simulink model "EngineSpeed_harness"  (Simulink 7.7)
settings: Solver=FixedStepDiscrete  SolverMode=SingleTasking  StartTime=0.0  StopTime=100  FixedStep=.01  RelTol=1e-3
InitFcn:
  | if signalbuilder('EngineSpeed_harness/Signal_Builder','activegroup') == 1
  |   CD_ENGINE_SPEED_FUNCTION.DataType = 'uint8';
  |   CD_ENGINE_SPEED_FUNCTION.Value = 255;
  | else
  |   CD_ENGINE_SPEED_FUNCTION.DataType = 'uint8';
  |   CD_ENGINE_SPEED_FUNCTION.Value = 0;
  | end
  | 
  | if signalbuilder('EngineSpeed_harness/Signal_Builder','activegroup') == 4
  |   CD_SHUTDOWN_FUNCTION.DataType = 'uint8';
  |   CD_SHUTDOWN_FUNCTION.Value = 255;
  | else
  |   CD_SHUTDOWN_FUNCTION.DataType = 'uint8';
  |   CD_SHUTDOWN_FUNCTION.Value = 0;
  | end
  | 
  | if signalbuilder('EngineSpeed_harness/Signal_Builder','activegroup') == 6
  |   CD_EOP_FUNCTION.DataType = 'uint8';
  |   CD_EOP_FUNCTION.Value = 0;
  | else
  |   CD_EOP_FUNCTION.DataType = 'uint8';
  |   CD_EOP_FUNCTION.Value = 1;
  | end
  | 
  | if (signalbuilder('EngineSpeed_harness/Signal_Builder','activegroup') == 6 || signalbuilder('EngineSpeed_harness/Signal_Builder','activegroup') == 7)
  |   CD_ENGINE_SPEED_DEBOUNCE_NO_SIGNAL.DataType = 'uint16';
  |   CD_ENGINE_SPEED_DEBOUNCE_NO_SIGNAL.Value = 100;
  |   CD_ENGINE_SPEED_DEBOUNCE_NORMAL.DataType = 'uint16';
  |   CD_ENGINE_SPEED_DEBOUNCE_NORMAL.Value = 50;
  | else
  |   CD_ENGINE_SPEED_DEBOUNCE_NO_SIGNAL.DataType = 'uint16';
  |   CD_ENGINE_SPEED_DEBOUNCE_NO_SIGNAL.Value = 3000;
  |   CD_ENGINE_SPEED_DEBOUNCE_NORMAL.DataType = 'uint16';
  |   CD_ENGINE_SPEED_DEBOUNCE_NORMAL.Value = 500;
  | end
  | 
  | if signalbuilder('EngineSpeed_harness/Signal_Builder','activegroup') == 9
  |   CD_ECU_FUNCTION.DataType = 'uint8';
  |   CD_ECU_FUNCTION.Value = 0;
  | else
  |   CD_ECU_FUNCTION.DataType = 'uint8';
  |   CD_ECU_FUNCTION.Value = 255;
  | end
  | 
  | if signalbuilder('EngineSpeed_harness/Signal_Builder','activegroup') == 14
  |   CD_ECU_FUNCTION.DataType = 'uint8';
  |   CD_ECU_FUNCTION.Value = 1;
  | end
undefined symbols (not defined in the file): CD_ENGINE_RPM_FACTOR, CD_ENGINE_SPEED_FILTER_FAST_VALUE, CD_ENGINE_SPEED_FILTER_SLOW_VALUE, CD_ENGINE_SPEED_RUNNING, CD_FLYWHEEL_TEETH, NON_FUNCTIONAL, PERIOD_COUNTS_PER_SECOND, sigbuilder_block, srate
libraries: simulink x2
CloseFcn:
  | rtwprivate ssgencode ModelCloseRequest sle_main_controller
settings Model: Creator=spencermindeman  LastModifiedBy=aliebel  CovMetricSettings=dcmw  CovForceBlockReductionOff=off  CovModelRefEnable=off
settings MATStruct: SampleTime=0.01  Offset=0  Priority=[1.0]
settings DataIOCC: LimitDataPoints=off  SaveOutput=off  SaveTime=off
settings OptimizationCC: BlockReduction=off  InlineParams=on  ExpressionFolding=off  StateBitsets=on  DataBitsets=on  UseTempVars=on  InitFltsAndDblsToZero=on  NoFixptDivByZeroProtection=on  EfficientFloat2IntCast=on  OptimizeModelRefInitCode=on
settings DebuggingCC: SaveWithParameterizedLinksMsg=none  MultiTaskDSMMsg=warning  MultiTaskCondExecSysMsg=none  IntegerOverflowMsg=none  ModelReferenceCSMismatchMessage=warning
settings HardwareCC: ProdBitPerInt=16  ProdBitPerPointer=16  ProdIntDivRoundTo=Floor  ProdEndianess=BigEndian  ProdWordSize=16  ProdHWDeviceType=Motorola HC12
settings ModelReferenceCC: ModelReferenceNumInstancesAllowed=Single
settings RTWCC: SystemTargetFile=ert.tlc  GenCodeOnly=on  TemplateMakefile=ert_default_tmf  Description=Real-Time Workshop Embedded Coder (no auto configuration)  GenerateReport=on  RetainRTWFile=on  ProcessScript=ert_make_rtw_hook  IncludeHyperlinkInReport=on  LaunchReport=on  IncludeERTFirstTime=on
settings RTWCC: CustomHeaderCode=|
  | #include "cpp_req_defines.h"
  | #include "hw_fin.h"
  | #include "cdata.h"
settings CodeAppCC: IgnoreCustomStorageClasses=off  DefineNamingRule=UpperCase
settings ERTTargetCC: TargetFcnLib=ansi_tfl_tmw.mat  FunctionExecutionProfile=off  MultiwordLength=2048  GenerateSampleERTMain=on  IncludeMdlTerminateFcn=off  SupportAbsoluteTime=off  SupportNonFinite=off  SupportComplex=off  PurelyIntegerCode=on  ERTCustomFileTemplate=gen_rtw_req_defines_h.tlc  GlobalDataDefinition=InSeparateSourceFile  GlobalDataReference=InSeparateHeaderFile  ConvertIfToSwitch=off

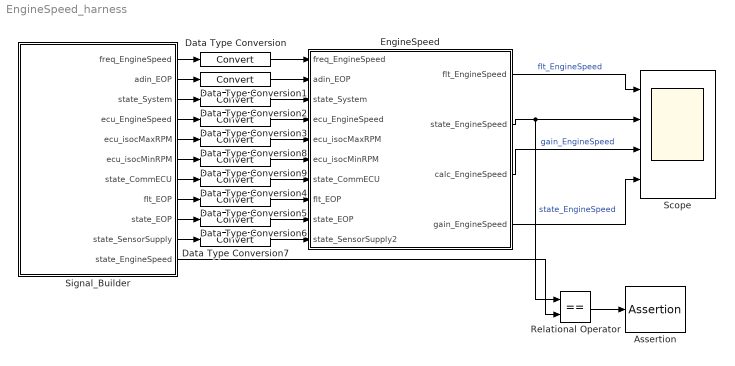
== system EngineSpeed_harness ==
  Assertion : Assertion  Enabled=off
  Data Type Conversion{,1..9} (10 alike) : DataTypeConversion
  EngineSpeed : Subsystem  TreatAsAtomicUnit=on  SystemSampleTime=srate  RTWFileName=mod_Inputs
      settings: RTWSystemCode=Function  RTWFcnNameOpts=Use subsystem name  RTWFileNameOpts=User specified
  Relational Operator : RelationalOperator  Operator===  OutDataTypeStr=boolean
  Scope : Scope  NumInputPorts=4
      settings: YMin=0~8~30~0  YMax=30~13~30~4  MaxDataPoints=50000
  Signal_Builder : Subsystem  Tag=STV Subsys  LoadFcn=sigbuilder_block('load');  StartFcn=sigbuilder_block('start');  StopFcn=sigbuilder_block('stop');  ClipboardFcn=sigbuilder_block('clipboard');  mask(Sigbuilder block){}
      mask help: Sigbuilder GUI
      mask init:
      | if ~strcmp(get_param(bdroot(gcbh),'SimulationStatus'),'stopped') tuvar = sigbuilder_block('maskInit'); end
      settings: CopyFcn=sigbuilder_block('copy');  DeleteFcn=sigbuilder_block('delete');  ModelCloseFcn=sigbuilder_block('modelClose');  PreSaveFcn=sigbuilder_block('preSave');  NameChangeFcn=sigbuilder_block('namechange');  OpenFcn=sigbuilder_block('open',[39.75 48.75 1278 690.75 ]);  CloseFcn=sigbuilder_block('close');
      mask Display: plot(0,0,100,100,[10,10,40,40,10],[80,20,20,80,80],[40,10],[50,50], [40,27,10],[65,72,56],[40,25,25,10],[28,28,43,43]);
  wires:
  Data Type Conversion/1 -> EngineSpeed/1(freq_EngineSpeed)
  Data Type Conversion1/1 -> EngineSpeed/2(adin_EOP)
  Data Type Conversion2/1 -> EngineSpeed/3(state_System)
  Signal_Builder/1(freq_EngineSpeed) -> Data Type Conversion/1
  Data Type Conversion3/1 -> EngineSpeed/4(ecu_EngineSpeed)
  Relational Operator/1 -> Assertion/1
  Signal_Builder/11(state_EngineSpeed) -> Relational Operator/2
  Data Type Conversion4/1 -> EngineSpeed/7(state_CommECU)
  Signal_Builder/2(adin_EOP) -> Data Type Conversion1/1
  Signal_Builder/3(state_System) -> Data Type Conversion2/1
  Signal_Builder/4(ecu_EngineSpeed) -> Data Type Conversion3/1
  Signal_Builder/7(state_CommECU) -> Data Type Conversion4/1
  Signal_Builder/8(flt_EOP) -> Data Type Conversion5/1
  Signal_Builder/9(state_EOP) -> Data Type Conversion6/1
  Data Type Conversion5/1 -> EngineSpeed/8(flt_EOP)
  Data Type Conversion6/1 -> EngineSpeed/9(state_EOP)
  EngineSpeed/1(flt_EngineSpeed) -> Scope/1  "flt_EngineSpeed"
  EngineSpeed/2(state_EngineSpeed) -> Scope/2, Relational Operator/1  "state_EngineSpeed"
  EngineSpeed/3(calc_EngineSpeed) -> Scope/3  "gain_EngineSpeed"
  Signal_Builder/10(state_SensorSupply) -> Data Type Conversion7/1
  Data Type Conversion7/1 -> EngineSpeed/10(state_SensorSupply2)
  EngineSpeed/4(gain_EngineSpeed) -> Scope/4
  Signal_Builder/5(ecu_isocMaxRPM) -> Data Type Conversion8/1
  Signal_Builder/6(ecu_isocMinRPM) -> Data Type Conversion9/1
  Data Type Conversion8/1 -> EngineSpeed/5(ecu_isocMaxRPM)
  Data Type Conversion9/1 -> EngineSpeed/6(ecu_isocMinRPM)

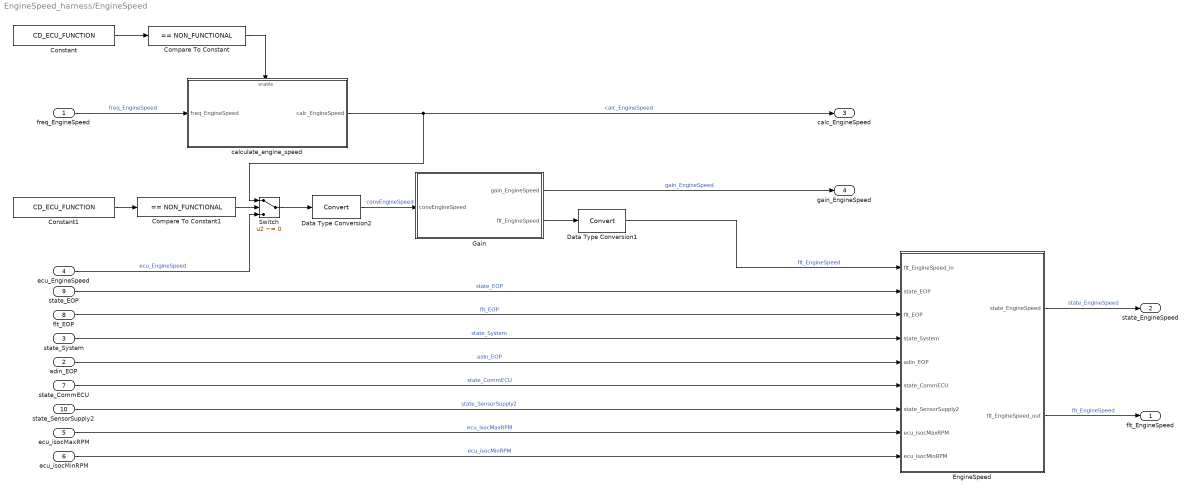
== system EngineSpeed_harness/EngineSpeed ==
  freq_EngineSpeed : Inport
  adin_EOP : Inport  Port=2
  state_System : Inport  Port=3
  ecu_EngineSpeed : Inport  Port=4
  ecu_isocMaxRPM : Inport  Port=5
  ecu_isocMinRPM : Inport  Port=6
  state_CommECU : Inport  Port=7
  flt_EOP : Inport  Port=8
  state_EOP : Inport  Port=9
  state_SensorSupply2 : Inport  Port=10
  Compare To Constant : simulink/Logic and Bit Operations/Compare To Constant  SystemSampleTime=-1  relop===  const=NON_FUNCTIONAL  LogicOutDataTypeMode=boolean  ZeroCross=off
  Compare To Constant1 : simulink/Logic and Bit Operations/Compare To Constant  SystemSampleTime=-1  relop===  const=NON_FUNCTIONAL  LogicOutDataTypeMode=boolean  ZeroCross=off
  Constant : Constant  Value=CD_ECU_FUNCTION  OutDataTypeStr=uint8
  Constant1 : Constant  Value=CD_ECU_FUNCTION  OutDataTypeStr=uint8
  Data Type Conversion1 : DataTypeConversion
  Data Type Conversion2 : DataTypeConversion
  EngineSpeed : Stateflow chart  TreatAsAtomicUnit=on
  Gain : Stateflow chart  TreatAsAtomicUnit=on
  Switch : Switch  Criteria=u2 ~= 0
  calculate_engine_speed : Subsystem
  flt_EngineSpeed : Outport  OutDataTypeStr=uint16
  state_EngineSpeed : Outport  Port=2  OutDataTypeStr=uint8
  calc_EngineSpeed : Outport  Port=3  OutDataTypeStr=uint16
  gain_EngineSpeed : Outport  Port=4
  wires:
  adin_EOP/1 -> EngineSpeed/5(adin_EOP)  "adin_EOP"
  state_System/1 -> EngineSpeed/4(state_System)  "state_System"
  state_EOP/1 -> EngineSpeed/2(state_EOP)  "state_EOP"
  EngineSpeed/1(state_EngineSpeed) -> state_EngineSpeed/1  "state_EngineSpeed"
  flt_EOP/1 -> EngineSpeed/3(flt_EOP)  "flt_EOP"
  state_CommECU/1 -> EngineSpeed/6(state_CommECU)  "state_CommECU"
  freq_EngineSpeed/1 -> calculate_engine_speed/1(freq_EngineSpeed)  "freq_EngineSpeed"
  Data Type Conversion1/1 -> EngineSpeed/1(flt_EngineSpeed_in)  "flt_EngineSpeed"
  state_SensorSupply2/1 -> EngineSpeed/7(state_SensorSupply2)  "state_SensorSupply2"
  Gain/2(flt_EngineSpeed) -> Data Type Conversion1/1
  Data Type Conversion2/1 -> Gain/1(convEngineSpeed)  "convEngineSpeed"
  Gain/1(gain_EngineSpeed) -> gain_EngineSpeed/1  "gain_EngineSpeed"
  calculate_engine_speed/1(calc_EngineSpeed) -> Switch/1, calc_EngineSpeed/1  "calc_EngineSpeed"
  Switch/1 -> Data Type Conversion2/1
  Constant/1 -> Compare To Constant/1
  Compare To Constant/1 -> calculate_engine_speed/Enable
  Constant1/1 -> Compare To Constant1/1
  Compare To Constant1/1 -> Switch/2
  ecu_EngineSpeed/1 -> Switch/3  "ecu_EngineSpeed"
  EngineSpeed/2(flt_EngineSpeed_out) -> flt_EngineSpeed/1  "flt_EngineSpeed"
  ecu_isocMaxRPM/1 -> EngineSpeed/8(ecu_isocMaxRPM)  "ecu_isocMaxRPM"
  ecu_isocMinRPM/1 -> EngineSpeed/9(ecu_isocMinRPM)  "ecu_isocMinRPM"

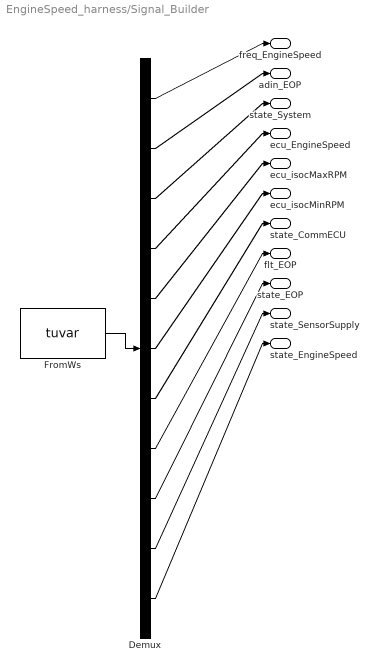
== system EngineSpeed_harness/Signal_Builder ==
  Demux : Demux  Tag=STV Demux  Outputs=11
  FromWs : FromWorkspace  Tag=STV FromWs  VariableName=tuvar  SampleTime=0  SigBuilderData=DataTag0  VnvData=DataTag1
      SigBuilderData=|
      | common.afterFinalStr = 'Extrapolate'
      | common.sampleTime = 0
      | dataSet(1).timeRange = [0 100]
      | dataSet(1).name = 'T1-NONFUNC'
      | dataSet(2).timeRange = [0 100]
      | dataSet(2).name = 'T2-NORMAL'
      | dataSet(3).timeRange = [0 100]
      | dataSet(3).name = 'T3-OOR'
      | dataSet(4).timeRange = [0 100]
      | dataSet(4).name = 'T4-EX HIGH'
      | dataSet(5).timeRange = [0 100]
      | dataSet(5).name = 'T5-Shutdown'
      | dataSet(6).timeRange = [0 100]
      | dataSet(6).name = 'T6-No Sig Sender'
      | dataSet(7).timeRange = [0 100]
      | dataSet(7).name = 'T7-No Sig Switch'
      | dataSet(8).timeRange = [0 100]
      | dataSet(8).name = 'T8-SystemState'
      | dataSet(9).timeRange = [0 100]
      | dataSet(9).name = 'T9-ECU'
      | dataSet(10).timeRange = [0 100]
      | dataSet(10).name = 'NORMAL1'
      | dataSet(11).timeRange = [0 100]
      | dataSet(11).name = 'NORMAL2'
      | dataSet(12).timeRange = [0 100]
      | dataSet(12).name = 'SystemState1'
      | dataSet(13).timeRange = [0 100]
      | dataSet(13).name = 'SystemState2'
      | dataSet(14).timeRange = [0 100]
      | dataSet(14).name = 'T14-ECU Invalid'
      | sbobj.Groups(1).Name = 'T1-NONFUNC'
      | sbobj.Groups(1).Signals(1).Name = 'freq_EngineSpeed'
      | sbobj.Groups(1).Signals(1).XData = [0 27.8 28.2 62.2 62.2 100]
      | sbobj.Groups(1).Signals(1).YData = [60000 60000 591 591 60500 60000]
      | sbobj.Groups(1).Signals(2).Name = 'adin_EOP'
      | sbobj.Groups(1).Signals(2).XData = [0 40 40 70 70 100]
      | sbobj.Groups(1).Signals(2).YData = [0 0 1000 1000 0 0]
      | sbobj.Groups(1).Signals(3).Name = 'state_System'
      | sbobj.Groups(1).Signals(3).XData = [0 100]
      | sbobj.Groups(1).Signals(3).YData = [1 1]
      | sbobj.Groups(1).Signals(4).Name = 'ecu_EngineSpeed'
      | sbobj.Groups(1).Signals(4).XData = [0 100]
      | sbobj.Groups(1).Signals(4).YData = [0 0]
      | sbobj.Groups(1).Signals(5).Name = 'ecu_isocMaxRPM'
      | sbobj.Groups(1).Signals(5).XData = [0 100]
      | sbobj.Groups(1).Signals(5).YData = [0 0]
      | sbobj.Groups(1).Signals(6).Name = 'ecu_isocMinRPM'
      | sbobj.Groups(1).Signals(6).XData = [0 100]
      | sbobj.Groups(1).Signals(6).YData = [0 0]
      | sbobj.Groups(1).Signals(7).Name = 'state_CommECU'
      | sbobj.Groups(1).Signals(7).XData = [0 100]
      | sbobj.Groups(1).Signals(7).YData = [0 0]
      | sbobj.Groups(1).Signals(8).Name = 'flt_EOP'
      | sbobj.Groups(1).Signals(8).XData = [0 18.2 18.2 19.4 19.4 21 21 32.6 32.6 33 33 36.6 36.6 48.4 48.4 100]
      | sbobj.Groups(1).Signals(8).YData = [0 0 25 25 0.5 0.5 25 25 0.5 0.5 25 25 0 0 25 25]
      | sbobj.Groups(1).Signals(9).Name = 'state_EOP'
      | sbobj.Groups(1).Signals(9).XData = [0 59.8 59.8 70.8 70.8 100]
      | sbobj.Groups(1).Signals(9).YData = [8 8 10 10 8 8]
      | sbobj.Groups(1).Signals(10).Name = 'state_SensorSupply'
      | sbobj.Groups(1).Signals(10).XData = [0 100]
      | sbobj.Groups(1).Signals(10).YData = [0 0]
      | sbobj.Groups(1).Signals(11).Name = 'state_EngineSpeed'
      | sbobj.Groups(1).Signals(11).XData = [0 100]
      | sbobj.Groups(1).Signals(11).YData = [8 8]
      | sbobj.Groups(2).Name = 'T2-NORMAL'
      | sbobj.Groups(2).Signals(1).Name = 'freq_EngineSpeed'
      | sbobj.Groups(2).Signals(1).XData = [0 39.7 100]
      | sbobj.Groups(2).Signals(1).YData = [1000 692 1000]
      | sbobj.Groups(2).Signals(2).Name = 'adin_EOP'
      | sbobj.Groups(2).Signals(2).XData = [0 100]
      | sbobj.Groups(2).Signals(2).YData = [0 0]
      | sbobj.Groups(2).Signals(3).Name = 'state_System'
      | sbobj.Groups(2).Signals(3).XData = [0 100]
      | sbobj.Groups(2).Signals(3).YData = [1 1]
      | sbobj.Groups(2).Signals(4).Name = 'ecu_EngineSpeed'
      | sbobj.Groups(2).Signals(4).XData = [0 100]
      | sbobj.Groups(2).Signals(4).YData = [0 0]
      | sbobj.Groups(2).Signals(5).Name = 'ecu_isocMaxRPM'
      | sbobj.Groups(2).Signals(5).XData = [0 100]
      | sbobj.Groups(2).Signals(5).YData = [0 0]
      | sbobj.Groups(2).Signals(6).Name = 'ecu_isocMinRPM'
      | sbobj.Groups(2).Signals(6).XData = [0 100]
      | sbobj.Groups(2).Signals(6).YData = [0 0]
      | sbobj.Groups(2).Signals(7).Name = 'state_CommECU'
      | sbobj.Groups(2).Signals(7).XData = [0 100]
      | sbobj.Groups(2).Signals(7).YData = [0 0]
      | sbobj.Groups(2).Signals(8).Name = 'flt_EOP'
      | sbobj.Groups(2).Signals(8).XData = [0 100]
      | sbobj.Groups(2).Signals(8).YData = [20 20]
      | sbobj.Groups(2).Signals(9).Name = 'state_EOP'
      | sbobj.Groups(2).Signals(9).XData = [0 100]
      | sbobj.Groups(2).Signals(9).YData = [8 8]
      | sbobj.Groups(2).Signals(10).Name = 'state_SensorSupply'
      | sbobj.Groups(2).Signals(10).XData = [0 100]
      | sbobj.Groups(2).Signals(10).YData = [8 8]
      | sbobj.Groups(2).Signals(11).Name = 'state_EngineSpeed'
      | sbobj.Groups(2).Signals(11).XData = [0 100]
      | sbobj.Groups(2).Signals(11).YData = [8 8]
      | sbobj.Groups(3).Name = 'T3-OOR'
      | sbobj.Groups(3).Signals(1).Name = 'freq_EngineSpeed'
      | sbobj.Groups(3).Signals(1).XData = [0 19.8 46.8 46.8 47.4 47.4 50.2 54.8 54.8 55 55 100]
      | sbobj.Groups(3).Signals(1).YData = [1000 1000 289.473684211 1020 980 247.368421053 200 198.152610442 1020 1020 196.546184739 180]
      | sbobj.Groups(3).Signals(2).Name = 'adin_EOP'
      | sbobj.Groups(3).Signals(2).XData = [0 100]
      | sbobj.Groups(3).Signals(2).YData = [0 0]
      | sbobj.Groups(3).Signals(3).Name = 'state_System'
      | sbobj.Groups(3).Signals(3).XData = [0 100]
      | sbobj.Groups(3).Signals(3).YData = [1 1]
      | sbobj.Groups(3).Signals(4).Name = 'ecu_EngineSpeed'
      | sbobj.Groups(3).Signals(4).XData = [0 100]
      | sbobj.Groups(3).Signals(4).YData = [0 0]
      | sbobj.Groups(3).Signals(5).Name = 'ecu_isocMaxRPM'
      | sbobj.Groups(3).Signals(5).XData = [0 100]
      | sbobj.Groups(3).Signals(5).YData = [0 0]
      | sbobj.Groups(3).Signals(6).Name = 'ecu_isocMinRPM'
      | sbobj.Groups(3).Signals(6).XData = [0 100]
      | sbobj.Groups(3).Signals(6).YData = [0 0]
      | sbobj.Groups(3).Signals(7).Name = 'state_CommECU'
      | sbobj.Groups(3).Signals(7).XData = [0 100]
      | sbobj.Groups(3).Signals(7).YData = [0 0]
      | sbobj.Groups(3).Signals(8).Name = 'flt_EOP'
      | sbobj.Groups(3).Signals(8).XData = [0 100]
      | sbobj.Groups(3).Signals(8).YData = [20 20]
      | sbobj.Groups(3).Signals(9).Name = 'state_EOP'
      | sbobj.Groups(3).Signals(9).XData = [0 100]
      | sbobj.Groups(3).Signals(9).YData = [8 8]
      | sbobj.Groups(3).Signals(10).Name = 'state_SensorSupply'
      | sbobj.Groups(3).Signals(10).XData = [0 100]
      | sbobj.Groups(3).Signals(10).YData = [8 8]
      | sbobj.Groups(3).Signals(11).Name = 'state_EngineSpeed'
      | sbobj.Groups(3).Signals(11).XData = [0 37.26 37.26 37.97 37.97 38.99 38.99 47.32 47.32 50.49 50.49 100]
      | sbobj.Groups(3).Signals(11).YData = [8 8 10 10 11 11 15 15 8 8 18 18]
      | sbobj.Groups(4).Name = 'T4-EX HIGH'
      | sbobj.Groups(4).Signals(1).Name = 'freq_EngineSpeed'
      | sbobj.Groups(4).Signals(1).XData = [0 29.6 40 40.2 40.2 40.3 40.3 45.9 45.9 46 46 49.6 49.6 49.7 49.7 51.9 51.9 52 52 53.8 53.8 54.6 55.6 55.6 64.7 64.7 64.8 64.8 79.8 100]
      | sbobj.Groups(4).Signals(1).YData = [1000 1000 550 550 800 800 500 500 800 800 500 500 420 420 500 500 400 400 500 500 490 490 490 420 420 740 680 420 420 420]
      | sbobj.Groups(4).Signals(2).Name = 'adin_EOP'
      | sbobj.Groups(4).Signals(2).XData = [0 100]
      | sbobj.Groups(4).Signals(2).YData = [0 0]
      | sbobj.Groups(4).Signals(3).Name = 'state_System'
      | sbobj.Groups(4).Signals(3).XData = [0 100]
      | sbobj.Groups(4).Signals(3).YData = [1 1]
      | sbobj.Groups(4).Signals(4).Name = 'ecu_EngineSpeed'
      | sbobj.Groups(4).Signals(4).XData = [0 100]
      | sbobj.Groups(4).Signals(4).YData = [0 0]
      | sbobj.Groups(4).Signals(5).Name = 'ecu_isocMaxRPM'
      | sbobj.Groups(4).Signals(5).XData = [0 100]
      | sbobj.Groups(4).Signals(5).YData = [0 0]
      | sbobj.Groups(4).Signals(6).Name = 'ecu_isocMinRPM'
      | sbobj.Groups(4).Signals(6).XData = [0 100]
      | sbobj.Groups(4).Signals(6).YData = [0 0]
      | sbobj.Groups(4).Signals(7).Name = 'state_CommECU'
      | sbobj.Groups(4).Signals(7).XData = [0 100]
      | sbobj.Groups(4).Signals(7).YData = [0 0]
      | sbobj.Groups(4).Signals(8).Name = 'flt_EOP'
      | sbobj.Groups(4).Signals(8).XData = [0 100]
      | sbobj.Groups(4).Signals(8).YData = [20 20]
      | sbobj.Groups(4).Signals(9).Name = 'state_EOP'
      | sbobj.Groups(4).Signals(9).XData = [0 100]
      | sbobj.Groups(4).Signals(9).YData = [8 8]
      | sbobj.Groups(4).Signals(10).Name = 'state_SensorSupply'
      | sbobj.Groups(4).Signals(10).XData = [0 100]
      | sbobj.Groups(4).Signals(10).YData = [8 8]
      | sbobj.Groups(4).Signals(11).Name = 'state_EngineSpeed'
      | sbobj.Groups(4).Signals(11).XData = [0 45.35 45.35 60.67 60.67 100]
      | sbobj.Groups(4).Signals(11).YData = [8 8 10 10 11 11]
      | sbobj.Groups(5).Name = 'T5-Shutdown'
      | sbobj.Groups(5).Signals(1).Name = 'freq_EngineSpeed'
      | sbobj.Groups(5).Signals(1).XData = [0 29.6 40 40.2 40.2 40.3 40.3 45.9 45.9 46 46 49.6 49.6 49.7 49.7 51.9 51.9 52 52 57.8 57.8 58.3 58.3 58.7 58.7 64.7 64.7 64.8 64.8 79.8 79.8 100]
      | sbobj.Groups(5).Signals(1).YData = [1000 1000 550 550 800 800 500 500 800 800 410 410 420 420 440 440 400 400 770 770 490 490 750 750 400 400 740 680 400 400 420 420]
      | sbobj.Groups(5).Signals(2).Name = 'adin_EOP'
      | sbobj.Groups(5).Signals(2).XData = [0 100]
      | sbobj.Groups(5).Signals(2).YData = [0 0]
      | sbobj.Groups(5).Signals(3).Name = 'state_System'
      | sbobj.Groups(5).Signals(3).XData = [0 100]
      | sbobj.Groups(5).Signals(3).YData = [1 1]
      | sbobj.Groups(5).Signals(4).Name = 'ecu_EngineSpeed'
      | sbobj.Groups(5).Signals(4).XData = [0 100]
      | sbobj.Groups(5).Signals(4).YData = [0 0]
      | sbobj.Groups(5).Signals(5).Name = 'ecu_isocMaxRPM'
      | sbobj.Groups(5).Signals(5).XData = [0 100]
      | sbobj.Groups(5).Signals(5).YData = [0 0]
      | sbobj.Groups(5).Signals(6).Name = 'ecu_isocMinRPM'
      | sbobj.Groups(5).Signals(6).XData = [0 100]
      | sbobj.Groups(5).Signals(6).YData = [0 0]
      | sbobj.Groups(5).Signals(7).Name = 'state_CommECU'
      | sbobj.Groups(5).Signals(7).XData = [0 100]
      | sbobj.Groups(5).Signals(7).YData = [0 0]
      | sbobj.Groups(5).Signals(8).Name = 'flt_EOP'
      | sbobj.Groups(5).Signals(8).XData = [0 100]
      | sbobj.Groups(5).Signals(8).YData = [20 20]
      | sbobj.Groups(5).Signals(9).Name = 'state_EOP'
      | sbobj.Groups(5).Signals(9).XData = [0 100]
      | sbobj.Groups(5).Signals(9).YData = [8 8]
      | sbobj.Groups(5).Signals(10).Name = 'state_SensorSupply'
      | sbobj.Groups(5).Signals(10).XData = [0 100]
      | sbobj.Groups(5).Signals(10).YData = [8 8]
      | sbobj.Groups(5).Signals(11).Name = 'state_EngineSpeed'
      | sbobj.Groups(5).Signals(11).XData = [0 45.35 45.35 51.04 51.04 57.04 57.04 63.78 63.78 74.84 74.84 100]
      | sbobj.Groups(5).Signals(11).YData = [8 8 10 10 11 11 8 8 11 11 15 15]
      | sbobj.Groups(6).Name = 'T6-No Sig Sender'
      | sbobj.Groups(6).Signals(1).Name = 'freq_EngineSpeed'
      | sbobj.Groups(6).Signals(1).XData = [0 82.4 82.4 100]
      | sbobj.Groups(6).Signals(1).YData = [60000 60000 3000 3000]
      | sbobj.Groups(6).Signals(2).Name = 'adin_EOP'
      | sbobj.Groups(6).Signals(2).XData = [0 100]
      | sbobj.Groups(6).Signals(2).YData = [0 0]
      | sbobj.Groups(6).Signals(3).Name = 'state_System'
      | sbobj.Groups(6).Signals(3).XData = [0 100]
      | sbobj.Groups(6).Signals(3).YData = [1 1]
      | sbobj.Groups(6).Signals(4).Name = 'ecu_EngineSpeed'
      | sbobj.Groups(6).Signals(4).XData = [0 100]
      | sbobj.Groups(6).Signals(4).YData = [0 0]
      | sbobj.Groups(6).Signals(5).Name = 'ecu_isocMaxRPM'
      | sbobj.Groups(6).Signals(5).XData = [0 100]
      | sbobj.Groups(6).Signals(5).YData = [0 0]
      | sbobj.Groups(6).Signals(6).Name = 'ecu_isocMinRPM'
      | sbobj.Groups(6).Signals(6).XData = [0 100]
      | sbobj.Groups(6).Signals(6).YData = [0 0]
      | sbobj.Groups(6).Signals(7).Name = 'state_CommECU'
      | sbobj.Groups(6).Signals(7).XData = [0 100]
      | sbobj.Groups(6).Signals(7).YData = [0 0]
      | sbobj.Groups(6).Signals(8).Name = 'flt_EOP'
      | sbobj.Groups(6).Signals(8).XData = [0 18.2 18.2 19.4 19.4 21 21 32.6 32.6 33 33 36.6 36.6 48.4 48.4 100]
      | sbobj.Groups(6).Signals(8).YData = [0 0 25 25 0.5 0.5 25 25 0.5 0.5 25 25 0 0 25 25]
      | sbobj.Groups(6).Signals(9).Name = 'state_EOP'
      | sbobj.Groups(6).Signals(9).XData = [0 45.8 45.8 49.3 49.3 59.8 59.8 70.8 70.8 100]
      | sbobj.Groups(6).Signals(9).YData = [8 8 10 10 8 8 10 10 8 8]
      | sbobj.Groups(6).Signals(10).Name = 'state_SensorSupply'
      | sbobj.Groups(6).Signals(10).XData = [0 69.2 69.2 75.4 75.4 79.8 79.8 81.8 81.8 100]
      | sbobj.Groups(6).Signals(10).YData = [8 8 22 22 8 8 22 22 8 8]
      | sbobj.Groups(6).Signals(11).Name = 'state_EngineSpeed'
      | sbobj.Groups(6).Signals(11).XData = [0 19.21 19.21 19.91 19.91 22.01 22.01 37.11 37.11 50.31 50.31 60.31 60.31 76.41 76.41 80.32 80.32 100]
      | sbobj.Groups(6).Signals(11).YData = [8 8 13 13 8 8 13 13 8 8 13 13 8 8 13 13 8 8]
      | sbobj.Groups(7).Name = 'T7-No Sig Switch'
      | sbobj.Groups(7).Signals(1).Name = 'freq_EngineSpeed'
      | sbobj.Groups(7).Signals(1).XData = [0 82.4 82.4 100]
      | sbobj.Groups(7).Signals(1).YData = [60000 60000 3000 3000]
      | sbobj.Groups(7).Signals(2).Name = 'adin_EOP'
      | sbobj.Groups(7).Signals(2).XData = [0 40 40 70 70 75.1 75.1 78.6 78.6 100]
      | sbobj.Groups(7).Signals(2).YData = [0 0 1000 1000 0 0 990 990 0 0]
      | sbobj.Groups(7).Signals(3).Name = 'state_System'
      | sbobj.Groups(7).Signals(3).XData = [0 100]
      | sbobj.Groups(7).Signals(3).YData = [1 1]
      | sbobj.Groups(7).Signals(4).Name = 'ecu_EngineSpeed'
      | sbobj.Groups(7).Signals(4).XData = [0 100]
      | sbobj.Groups(7).Signals(4).YData = [0 0]
      | sbobj.Groups(7).Signals(5).Name = 'ecu_isocMaxRPM'
      | sbobj.Groups(7).Signals(5).XData = [0 100]
      | sbobj.Groups(7).Signals(5).YData = [0 0]
      | sbobj.Groups(7).Signals(6).Name = 'ecu_isocMinRPM'
      | sbobj.Groups(7).Signals(6).XData = [0 100]
      | sbobj.Groups(7).Signals(6).YData = [0 0]
      | sbobj.Groups(7).Signals(7).Name = 'state_CommECU'
      | sbobj.Groups(7).Signals(7).XData = [0 100]
      | sbobj.Groups(7).Signals(7).YData = [0 0]
      | sbobj.Groups(7).Signals(8).Name = 'flt_EOP'
      | sbobj.Groups(7).Signals(8).XData = [0 18.2 18.2 19.4 19.4 21 21 32.6 32.6 33 33 36.6 36.6 48.4 48.4 100]
      | sbobj.Groups(7).Signals(8).YData = [0 0 25 25 0.5 0.5 25 25 0.5 0.5 25 25 0 0 25 25]
      | sbobj.Groups(7).Signals(9).Name = 'state_EOP'
      | sbobj.Groups(7).Signals(9).XData = [0 9.8 9.8 35.4 35.4 42.3 42.3 59.8 59.8 70.8 70.8 100]
      | sbobj.Groups(7).Signals(9).YData = [9 9 8 8 9 9 8 8 10 10 8 8]
      | sbobj.Groups(7).Signals(10).Name = 'state_SensorSupply'
      | sbobj.Groups(7).Signals(10).XData = [0 100]
      | sbobj.Groups(7).Signals(10).YData = [8 8]
      | sbobj.Groups(7).Signals(11).Name = 'state_EngineSpeed'
      | sbobj.Groups(7).Signals(11).XData = [0 43.31 43.31 60.31 60.31 76.11 76.11 79.11 79.11 100]
      | sbobj.Groups(7).Signals(11).YData = [8 8 13 13 8 8 13 13 8 8]
      | sbobj.Groups(8).Name = 'T8-SystemState'
      | sbobj.Groups(8).Signals(1).Name = 'freq_EngineSpeed'
      | sbobj.Groups(8).Signals(1).XData = [0 39.7 100]
      | sbobj.Groups(8).Signals(1).YData = [1000 692 1000]
      | sbobj.Groups(8).Signals(2).Name = 'adin_EOP'
      | sbobj.Groups(8).Signals(2).XData = [0 100]
      | sbobj.Groups(8).Signals(2).YData = [0 0]
      | sbobj.Groups(8).Signals(3).Name = 'state_System'
      | sbobj.Groups(8).Signals(3).XData = [0 14.8 14.8 49.8 49.8 70 70 100]
      | sbobj.Groups(8).Signals(3).YData = [0 0 1 1 0 0 1 1]
      | sbobj.Groups(8).Signals(4).Name = 'ecu_EngineSpeed'
      | sbobj.Groups(8).Signals(4).XData = [0 100]
      | sbobj.Groups(8).Signals(4).YData = [0 0]
      | sbobj.Groups(8).Signals(5).Name = 'ecu_isocMaxRPM'
      | sbobj.Groups(8).Signals(5).XData = [0 100]
      | sbobj.Groups(8).Signals(5).YData = [0 0]
      | sbobj.Groups(8).Signals(6).Name = 'ecu_isocMinRPM'
      | sbobj.Groups(8).Signals(6).XData = [0 100]
      | sbobj.Groups(8).Signals(6).YData = [0 0]
      | sbobj.Groups(8).Signals(7).Name = 'state_CommECU'
      | sbobj.Groups(8).Signals(7).XData = [0 100]
      | sbobj.Groups(8).Signals(7).YData = [0 0]
      | sbobj.Groups(8).Signals(8).Name = 'flt_EOP'
      | sbobj.Groups(8).Signals(8).XData = [0 100]
      | sbobj.Groups(8).Signals(8).YData = [20 20]
      | sbobj.Groups(8).Signals(9).Name = 'state_EOP'
      | sbobj.Groups(8).Signals(9).XData = [0 100]
      | sbobj.Groups(8).Signals(9).YData = [8 8]
      | sbobj.Groups(8).Signals(10).Name = 'state_SensorSupply'
      | sbobj.Groups(8).Signals(10).XData = [0 100]
      | sbobj.Groups(8).Signals(10).YData = [8 8]
      | sbobj.Groups(8).Signals(11).Name = 'state_EngineSpeed'
      | sbobj.Groups(8).Signals(11).XData = [0 100]
      | sbobj.Groups(8).Signals(11).YData = [8 8]
      | sbobj.Groups(9).Name = 'T9-ECU'
      | sbobj.Groups(9).Signals(1).Name = 'freq_EngineSpeed'
      | sbobj.Groups(9).Signals(1).XData = [0 39.7 100]
      | sbobj.Groups(9).Signals(1).YData = [1000 692 1000]
      | sbobj.Groups(9).Signals(2).Name = 'adin_EOP'
      | sbobj.Groups(9).Signals(2).XData = [0 100]
      | sbobj.Groups(9).Signals(2).YData = [0 0]
      | sbobj.Groups(9).Signals(3).Name = 'state_System'
      | sbobj.Groups(9).Signals(3).XData = [0 100]
      | sbobj.Groups(9).Signals(3).YData = [1 1]
      | sbobj.Groups(9).Signals(4).Name = 'ecu_EngineSpeed'
      | sbobj.Groups(9).Signals(4).XData = [0 50.1 100]
      | sbobj.Groups(9).Signals(4).YData = [0 3000 0]
      | sbobj.Groups(9).Signals(5).Name = 'ecu_isocMaxRPM'
      | sbobj.Groups(9).Signals(5).XData = [0 100]
      | sbobj.Groups(9).Signals(5).YData = [0 0]
      | sbobj.Groups(9).Signals(6).Name = 'ecu_isocMinRPM'
      | sbobj.Groups(9).Signals(6).XData = [0 100]
      | sbobj.Groups(9).Signals(6).YData = [0 0]
      | sbobj.Groups(9).Signals(7).Name = 'state_CommECU'
      | sbobj.Groups(9).Signals(7).XData = [0 43.6 43.6 55.1 55.1 100]
      | sbobj.Groups(9).Signals(7).YData = [8 8 4 4 8 8]
      | sbobj.Groups(9).Signals(8).Name = 'flt_EOP'
      | sbobj.Groups(9).Signals(8).XData = [0 43.2 43.2 54.3 54.3 100]
      | sbobj.Groups(9).Signals(8).YData = [20 20 4 4 20 20]
      | sbobj.Groups(9).Signals(9).Name = 'state_EOP'
      | sbobj.Groups(9).Signals(9).XData = [0 100]
      | sbobj.Groups(9).Signals(9).YData = [8 8]
      | sbobj.Groups(9).Signals(10).Name = 'state_SensorSupply'
      | sbobj.Groups(9).Signals(10).XData = [0 100]
      | sbobj.Groups(9).Signals(10).YData = [8 8]
      | sbobj.Groups(9).Signals(11).Name = 'state_EngineSpeed'
      | sbobj.Groups(9).Signals(11).XData = [0 100]
      | sbobj.Groups(9).Signals(11).YData = [8 8]
      | sbobj.Groups(10).Name = 'NORMAL1'
      | sbobj.Groups(10).Signals(1).Name = 'freq_EngineSpeed'
      | sbobj.Groups(10).Signals(1).XData = [0 0.01 0.02 0.03 0.04 0.05 0.06 0.07 0.08 0.09 0.1 0.11 ... (1841 elements, 1x1841)]
      | sbobj.Groups(10).Signals(1).YData = [1028 1028 1021 1027 1020 1022 1028 1021 1021 1030 1024 1036 ... (1841 elements, 1x1841)]
      | sbobj.Groups(10).Signals(2).Name = 'adin_EOP'
      | sbobj.Groups(10).Signals(2).XData = [0 100]
      | sbobj.Groups(10).Signals(2).YData = [0 0]
      | sbobj.Groups(10).Signals(3).Name = 'state_System'
      | sbobj.Groups(10).Signals(3).XData = [0 100]
      | sbobj.Groups(10).Signals(3).YData = [1 1]
      | sbobj.Groups(10).Signals(4).Name = 'ecu_EngineSpeed'
      | sbobj.Groups(10).Signals(4).XData = [0 100]
      | sbobj.Groups(10).Signals(4).YData = [0 0]
      | sbobj.Groups(10).Signals(5).Name = 'ecu_isocMaxRPM'
      | sbobj.Groups(10).Signals(5).XData = [0 100]
      | sbobj.Groups(10).Signals(5).YData = [0 0]
      | sbobj.Groups(10).Signals(6).Name = 'ecu_isocMinRPM'
      | sbobj.Groups(10).Signals(6).XData = [0 100]
      | sbobj.Groups(10).Signals(6).YData = [0 0]
      | sbobj.Groups(10).Signals(7).Name = 'state_CommECU'
      | sbobj.Groups(10).Signals(7).XData = [0 100]
      | sbobj.Groups(10).Signals(7).YData = [0 0]
      | sbobj.Groups(10).Signals(8).Name = 'flt_EOP'
      | sbobj.Groups(10).Signals(8).XData = [0 100]
      | sbobj.Groups(10).Signals(8).YData = [20 20]
      | sbobj.Groups(10).Signals(9).Name = 'state_EOP'
      | sbobj.Groups(10).Signals(9).XData = [0 100]
      | sbobj.Groups(10).Signals(9).YData = [8 8]
      | sbobj.Groups(10).Signals(10).Name = 'state_SensorSupply'
      | sbobj.Groups(10).Signals(10).XData = [0 100]
      | sbobj.Groups(10).Signals(10).YData = [8 8]
      | sbobj.Groups(10).Signals(11).Name = 'state_EngineSpeed'
      | sbobj.Groups(10).Signals(11).XData = [0 100]
      | sbobj.Groups(10).Signals(11).YData = [8 8]
      | sbobj.Groups(11).Name = 'NORMAL2'
      | sbobj.Groups(11).Signals(1).Name = 'freq_EngineSpeed'
      | sbobj.Groups(11).Signals(1).XData = [0 0.01 0.02 0.03 0.04 0.05 0.06 0.07 0.08 0.09 0.1 0.11 ... (7018 elements, 1x7018)]
      | sbobj.Groups(11).Signals(1).YData = [1552 1552 1471 1355 1387 1292 1313 1313 1227 1188 1163 1178 ... (7018 elements, 1x7018)]
      | sbobj.Groups(11).Signals(2).Name = 'adin_EOP'
      | sbobj.Groups(11).Signals(2).XData = [0 100]
      | sbobj.Groups(11).Signals(2).YData = [0 0]
      | sbobj.Groups(11).Signals(3).Name = 'state_System'
      | sbobj.Groups(11).Signals(3).XData = [0 100]
      | sbobj.Groups(11).Signals(3).YData = [1 1]
      | sbobj.Groups(11).Signals(4).Name = 'ecu_EngineSpeed'
      | sbobj.Groups(11).Signals(4).XData = [0 100]
      | sbobj.Groups(11).Signals(4).YData = [0 0]
      | sbobj.Groups(11).Signals(5).Name = 'ecu_isocMaxRPM'
      | sbobj.Groups(11).Signals(5).XData = [0 100]
      | sbobj.Groups(11).Signals(5).YData = [0 0]
      | sbobj.Groups(11).Signals(6).Name = 'ecu_isocMinRPM'
      | sbobj.Groups(11).Signals(6).XData = [0 100]
      | sbobj.Groups(11).Signals(6).YData = [0 0]
      | sbobj.Groups(11).Signals(7).Name = 'state_CommECU'
      | sbobj.Groups(11).Signals(7).XData = [0 100]
      | sbobj.Groups(11).Signals(7).YData = [0 0]
      | sbobj.Groups(11).Signals(8).Name = 'flt_EOP'
      | sbobj.Groups(11).Signals(8).XData = [0 100]
      | sbobj.Groups(11).Signals(8).YData = [20 20]
      | sbobj.Groups(11).Signals(9).Name = 'state_EOP'
      | sbobj.Groups(11).Signals(9).XData = [0 100]
      | sbobj.Groups(11).Signals(9).YData = [8 8]
      | sbobj.Groups(11).Signals(10).Name = 'state_SensorSupply'
      | sbobj.Groups(11).Signals(10).XData = [0 100]
      | sbobj.Groups(11).Signals(10).YData = [8 8]
      | sbobj.Groups(11).Signals(11).Name = 'state_EngineSpeed'
      | sbobj.Groups(11).Signals(11).XData = [0 100]
      | sbobj.Groups(11).Signals(11).YData = [8 8]
      | sbobj.Groups(12).Name = 'SystemState1'
      | sbobj.Groups(12).Signals(1).Name = 'freq_EngineSpeed'
      | sbobj.Groups(12).Signals(1).XData = [0 0.02 0.04 0.06 0.08 0.1 0.12 0.14 0.16 0.18 0.2 0.22 ... (5001 elements, 1x5001)]
      | sbobj.Groups(12).Signals(1).YData = [1188 1163 1178 1131 1129 1111 1118 1123 1112 1130 1144 1155 ... (5001 elements, 1x5001)]
      | sbobj.Groups(12).Signals(2).Name = 'adin_EOP'
      | sbobj.Groups(12).Signals(2).XData = [0 100]
      | sbobj.Groups(12).Signals(2).YData = [0 0]
      | sbobj.Groups(12).Signals(3).Name = 'state_System'
      | sbobj.Groups(12).Signals(3).XData = [0 100]
      | sbobj.Groups(12).Signals(3).YData = [1 1]
      | sbobj.Groups(12).Signals(4).Name = 'ecu_EngineSpeed'
      | sbobj.Groups(12).Signals(4).XData = [0 100]
      | sbobj.Groups(12).Signals(4).YData = [0 0]
      | sbobj.Groups(12).Signals(5).Name = 'ecu_isocMaxRPM'
      | sbobj.Groups(12).Signals(5).XData = [0 100]
      | sbobj.Groups(12).Signals(5).YData = [0 0]
      | sbobj.Groups(12).Signals(6).Name = 'ecu_isocMinRPM'
      | sbobj.Groups(12).Signals(6).XData = [0 100]
      | sbobj.Groups(12).Signals(6).YData = [0 0]
      | sbobj.Groups(12).Signals(7).Name = 'state_CommECU'
      | sbobj.Groups(12).Signals(7).XData = [0 100]
      | sbobj.Groups(12).Signals(7).YData = [0 0]
      | sbobj.Groups(12).Signals(8).Name = 'flt_EOP'
      | sbobj.Groups(12).Signals(8).XData = [0 100]
      | sbobj.Groups(12).Signals(8).YData = [20 20]
      | sbobj.Groups(12).Signals(9).Name = 'state_EOP'
      | sbobj.Groups(12).Signals(9).XData = [0 100]
      | sbobj.Groups(12).Signals(9).YData = [8 8]
      | sbobj.Groups(12).Signals(10).Name = 'state_SensorSupply'
      | sbobj.Groups(12).Signals(10).XData = [0 100]
      | sbobj.Groups(12).Signals(10).YData = [8 8]
      | sbobj.Groups(12).Signals(11).Name = 'state_EngineSpeed'
      | sbobj.Groups(12).Signals(11).XData = [0 100]
      | sbobj.Groups(12).Signals(11).YData = [8 8]
      | sbobj.Groups(13).Name = 'SystemState2'
      | sbobj.Groups(13).Signals(1).Name = 'freq_EngineSpeed'
      | sbobj.Groups(13).Signals(1).XData = [0 0.01 0.02 0.03 0.04 0.05 0.06 0.07 0.08 0.09 0.1 0.11 ... (7012 elements, 1x7012)]
      | sbobj.Groups(13).Signals(1).YData = [1188 1163 1178 1131 1129 1111 1118 1123 1112 1130 1144 1155 ... (7012 elements, 1x7012)]
      | sbobj.Groups(13).Signals(2).Name = 'adin_EOP'
      | sbobj.Groups(13).Signals(2).XData = [0 100]
      | sbobj.Groups(13).Signals(2).YData = [0 0]
      | sbobj.Groups(13).Signals(3).Name = 'state_System'
      | sbobj.Groups(13).Signals(3).XData = [0 100]
      | sbobj.Groups(13).Signals(3).YData = [1 1]
      | sbobj.Groups(13).Signals(4).Name = 'ecu_EngineSpeed'
      | sbobj.Groups(13).Signals(4).XData = [0 100]
      | sbobj.Groups(13).Signals(4).YData = [0 0]
      | sbobj.Groups(13).Signals(5).Name = 'ecu_isocMaxRPM'
      | sbobj.Groups(13).Signals(5).XData = [0 100]
      | sbobj.Groups(13).Signals(5).YData = [0 0]
      | sbobj.Groups(13).Signals(6).Name = 'ecu_isocMinRPM'
      | sbobj.Groups(13).Signals(6).XData = [0 100]
      | sbobj.Groups(13).Signals(6).YData = [0 0]
      | sbobj.Groups(13).Signals(7).Name = 'state_CommECU'
      | sbobj.Groups(13).Signals(7).XData = [0 100]
      | sbobj.Groups(13).Signals(7).YData = [0 0]
      | sbobj.Groups(13).Signals(8).Name = 'flt_EOP'
      | sbobj.Groups(13).Signals(8).XData = [0 100]
      | sbobj.Groups(13).Signals(8).YData = [20 20]
      | sbobj.Groups(13).Signals(9).Name = 'state_EOP'
      | sbobj.Groups(13).Signals(9).XData = [0 100]
      | sbobj.Groups(13).Signals(9).YData = [8 8]
      | sbobj.Groups(13).Signals(10).Name = 'state_SensorSupply'
      | sbobj.Groups(13).Signals(10).XData = [0 100]
      | sbobj.Groups(13).Signals(10).YData = [8 8]
      | sbobj.Groups(13).Signals(11).Name = 'state_EngineSpeed'
      | sbobj.Groups(13).Signals(11).XData = [0 100]
      | sbobj.Groups(13).Signals(11).YData = [8 8]
      | sbobj.Groups(14).Name = 'T14-ECU Invalid'
      | sbobj.Groups(14).Signals(1).Name = 'freq_EngineSpeed'
      | sbobj.Groups(14).Signals(1).XData = [0 39.7 100]
      | sbobj.Groups(14).Signals(1).YData = [1000 692 1000]
      | sbobj.Groups(14).Signals(2).Name = 'adin_EOP'
      | sbobj.Groups(14).Signals(2).XData = [0 100]
      | sbobj.Groups(14).Signals(2).YData = [0 0]
      | sbobj.Groups(14).Signals(3).Name = 'state_System'
      | sbobj.Groups(14).Signals(3).XData = [0 100]
      | sbobj.Groups(14).Signals(3).YData = [1 1]
      | sbobj.Groups(14).Signals(4).Name = 'ecu_EngineSpeed'
      | sbobj.Groups(14).Signals(4).XData = [0 50.1 100]
      | sbobj.Groups(14).Signals(4).YData = [0 3000 0]
      | sbobj.Groups(14).Signals(5).Name = 'ecu_isocMaxRPM'
      | sbobj.Groups(14).Signals(5).XData = [0 1 1 5 5 6 6 11.1 11.1 14 14 17.7 17.7 21.9 21.9 23.8 23.8 100]
      | sbobj.Groups(14).Signals(5).YData = [2500 2500 1900 1900 2500 2500 1900 1900 2500 2500 3100 3100 2500 2500 3100 3100 2500 2500]
      | sbobj.Groups(14).Signals(6).Name = 'ecu_isocMinRPM'
      | sbobj.Groups(14).Signals(6).XData = [0 100]
      | sbobj.Groups(14).Signals(6).YData = [1000 1000]
      | sbobj.Groups(14).Signals(7).Name = 'state_CommECU'
      | sbobj.Groups(14).Signals(7).XData = [0 12 12 13 13 100]
      | sbobj.Groups(14).Signals(7).YData = [8 8 4 4 8 8]
      | sbobj.Groups(14).Signals(8).Name = 'flt_EOP'
      | sbobj.Groups(14).Signals(8).XData = [0 43.2 43.2 54.3 54.3 100]
      | sbobj.Groups(14).Signals(8).YData = [20 20 4 4 20 20]
      | sbobj.Groups(14).Signals(9).Name = 'state_EOP'
      | sbobj.Groups(14).Signals(9).XData = [0 100]
      | sbobj.Groups(14).Signals(9).YData = [8 8]
      | sbobj.Groups(14).Signals(10).Name = 'state_SensorSupply'
      | sbobj.Groups(14).Signals(10).XData = [0 100]
      | sbobj.Groups(14).Signals(10).YData = [8 8]
      | sbobj.Groups(14).Signals(11).Name = 'state_EngineSpeed'
      | sbobj.Groups(14).Signals(11).XData = [0 100]
      | sbobj.Groups(14).Signals(11).YData = [8 8]
  freq_EngineSpeed : Outport  Tag=STV Outport
  adin_EOP : Outport  Tag=STV Outport  Port=2
  state_System : Outport  Tag=STV Outport  Port=3
  ecu_EngineSpeed : Outport  Tag=STV Outport  Port=4
  ecu_isocMaxRPM : Outport  Tag=STV Outport  Port=5
  ecu_isocMinRPM : Outport  Tag=STV Outport  Port=6
  state_CommECU : Outport  Tag=STV Outport  Port=7
  flt_EOP : Outport  Tag=STV Outport  Port=8
  state_EOP : Outport  Tag=STV Outport  Port=9
  state_SensorSupply : Outport  Tag=STV Outport  Port=10
  state_EngineSpeed : Outport  Tag=STV Outport  Port=11
  wires:
  FromWs/1 -> Demux/1
  Demux/1 -> freq_EngineSpeed/1
  Demux/2 -> adin_EOP/1
  Demux/3 -> state_System/1
  Demux/4 -> ecu_EngineSpeed/1
  Demux/5 -> ecu_isocMaxRPM/1
  Demux/6 -> ecu_isocMinRPM/1
  Demux/7 -> state_CommECU/1
  Demux/8 -> flt_EOP/1
  Demux/9 -> state_EOP/1
  Demux/10 -> state_SensorSupply/1
  Demux/11 -> state_EngineSpeed/1

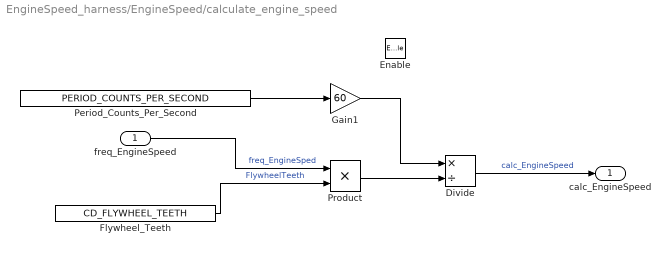
== system EngineSpeed_harness/EngineSpeed/calculate_engine_speed ==
  freq_EngineSpeed : Inport
  Enable : EnablePort  StatesWhenEnabling=reset
  Divide : Product  Inputs=*/  OutDataTypeStr=uint16
  Flywheel_Teeth : Constant  Value=CD_FLYWHEEL_TEETH  OutDataTypeStr=uint16
  Gain1 : Gain  Gain=60  ParamDataTypeStr=uint8  OutDataTypeStr=uint32
  Period_Counts_Per_Second : Constant  Value=PERIOD_COUNTS_PER_SECOND  OutDataTypeStr=uint32
  Product : Product  OutDataTypeStr=uint32  RndMeth=Zero
  calc_EngineSpeed : Outport  InitialOutput=[0]
  wires:
  Gain1/1 -> Divide/1
  Period_Counts_Per_Second/1 -> Gain1/1
  Divide/1 -> calc_EngineSpeed/1  "calc_EngineSpeed"
  Product/1 -> Divide/2
  Flywheel_Teeth/1 -> Product/2  "FlywheelTeeth"
  freq_EngineSpeed/1 -> Product/1  "freq_EngineSped"

== stateflow chart EngineSpeed/Gain ==
  state GAIN [parallel]
    settings: executionOrder=1
    state SLOW_FILTER
      du:gain_EngineSpeed = CD_ENGINE_SPEED_FILTER_SLOW_VALUE;
      SLOW_FILTER -> (junction 15) [order 1]
      (junction 15) -> (junction 17) [order 1] : [(flt_EngineSpeed > convEngineSpeed)]
      (junction 17) -> (junction 18) : {
          | change_EngineSpeed = flt_EngineSpeed - convEngineSpeed;
          | }
      (junction 15) -> (junction 16) [order 2] : {
          | change_EngineSpeed = convEngineSpeed - flt_EngineSpeed;
          | }
      (junction 18) -> (junction 16)
    state FAST_FILTER
      state FILTER [parallel]
        settings: executionOrder=2
        state FILTER_COUNT
          en:count_Factor = 0;
          du:count_Factor++;
        state FILTER
          du:gain_EngineSpeed = CD_ENGINE_SPEED_FILTER_FAST_VALUE;
        state FILTER1
          du:gain_EngineSpeed = 0;
        FILTER_COUNT -> GAIN.FAST_FILTER.FILTER.FILTER [order 1] : [(count_Factor > 1)...
            | || (convEngineSpeed < CD_ENGINE_SPEED_RUNNING)]
        (default) -> FILTER_COUNT
        GAIN.FAST_FILTER.FILTER.FILTER -> FILTER1 : [(convEngineSpeed == 0)]
        FILTER_COUNT -> FILTER1 [order 2] : [(convEngineSpeed == 0)]
        FILTER1 -> FILTER_COUNT : [(convEngineSpeed != 0)]
      state CHANGE [parallel]
        settings: executionOrder=1
        (junction 22) -> (junction 20)
        (junction 19) -> (junction 20) [order 2] : {
            | change_EngineSpeed = convEngineSpeed - flt_EngineSpeed;
            | }
        (junction 21) -> (junction 22) : {
            | change_EngineSpeed = flt_EngineSpeed - convEngineSpeed;
            | }
        (junction 19) -> (junction 21) [order 1] : [(flt_EngineSpeed > convEngineSpeed)]
        CHANGE -> (junction 19)
    FAST_FILTER -> SLOW_FILTER : [(change_EngineSpeed <= CD_ENGINE_RPM_FACTOR)...
        | && (convEngineSpeed >= CD_ENGINE_SPEED_RUNNING)]
    SLOW_FILTER -> FAST_FILTER [order 1] : [(change_EngineSpeed > CD_ENGINE_RPM_FACTOR)...
        | || (convEngineSpeed < CD_ENGINE_SPEED_RUNNING)]
    (default) -> SLOW_FILTER
  state FILTER [parallel]
    settings: executionOrder=2
    state INITIAL
      en:flt_EngineSpeed = convEngineSpeed;
    state LP_FILTER
      du:flt_EngineSpeed = (flt_EngineSpeed - ((flt_EngineSpeed - convEngineSpeed) >> gain_EngineSpeed));
    state LP_FILTER_GREATER
      du:flt_EngineSpeed = (flt_EngineSpeed + ((convEngineSpeed - flt_EngineSpeed) >> gain_EngineSpeed));
    INITIAL -> LP_FILTER [order 2]
    INITIAL -> LP_FILTER_GREATER [order 1] : [(convEngineSpeed > flt_EngineSpeed)]
    (default) -> INITIAL
    LP_FILTER -> LP_FILTER_GREATER : [(convEngineSpeed > flt_EngineSpeed)]
    LP_FILTER_GREATER -> LP_FILTER : [(convEngineSpeed <= flt_EngineSpeed)]
  data: convEngineSpeed input int16; gain_EngineSpeed output uint8; CD_ENGINE_RPM_FACTOR parameter uint8; CD_ENGINE_SPEED_FILTER_SLOW_VALUE parameter uint8; CD_ENGINE_SPEED_FILTER_FAST_VALUE parameter uint8; flt_EngineSpeed output fixdt(1,32,16); count_Factor local uint8; change_EngineSpeed local uint16; CD_ENGINE_SPEED_RUNNING parameter uint16

== stateflow chart EngineSpeed/EngineSpeed ==
  state SENSOR
    du:flt_EngineSpeed_out = flt_EngineSpeed_in;
    state OUT_OF_RANGE
      state DEBOUNCE
        en:debounceCount = 0;
        du:debounceCount++;
      state OUT_OF_RANGE
        en:state_EngineSpeed = OUT_OF_RANGE;
      SENSOR.OUT_OF_RANGE.DEBOUNCE -> SENSOR.OUT_OF_RANGE.OUT_OF_RANGE : [(debounceCount >= CD_ENGINE_SPEED_DEBOUNCE_OUT_OF_RANGE)...
          | || (state_EngineSpeed == OUT_OF_RANGE)]
      (default) -> SENSOR.OUT_OF_RANGE.DEBOUNCE
    state NORMAL
      state SHUTDOWN
        state DEBOUNCE
          en:debounceCount = 0;
          du:debounceCount++;
        state SHUTDOWN
          en:state_EngineSpeed = SHUTDOWN;
        SENSOR.NORMAL.SHUTDOWN.DEBOUNCE -> SENSOR.NORMAL.SHUTDOWN.SHUTDOWN : [(debounceCount >= CD_ENGINE_SPEED_DEBOUNCE_SHUTDOWN)]
        (default) -> SENSOR.NORMAL.SHUTDOWN.DEBOUNCE
      state EXTREMELY_HIGH
        state DEBOUNCE
          en:debounceCount = 0;
          du:debounceCount++;
        state EXTREMELY_HIGH
          en:state_EngineSpeed = EXTREMELY_HIGH;
        SENSOR.NORMAL.EXTREMELY_HIGH.DEBOUNCE -> SENSOR.NORMAL.EXTREMELY_HIGH.EXTREMELY_HIGH : [(debounceCount >= CD_ENGINE_SPEED_DEBOUNCE_EXTREMELY_HIGH)...
            | || (state_EngineSpeed == EXTREMELY_HIGH)]
        (default) -> SENSOR.NORMAL.EXTREMELY_HIGH.DEBOUNCE
      state HIGH
        state DEBOUNCE
          en:debounceCount = 0;
          du:debounceCount++;
        state HIGH
          en:state_EngineSpeed = HIGH;
        SENSOR.NORMAL.HIGH.DEBOUNCE -> SENSOR.NORMAL.HIGH.HIGH : [(debounceCount >= CD_ENGINE_SPEED_DEBOUNCE_HIGH)...
            | || (state_EngineSpeed == HIGH)]
        (default) -> SENSOR.NORMAL.HIGH.DEBOUNCE
      state NORMAL
        state DEBOUNCE
          en:debounceCount = 0;
          du:debounceCount++;
        state NORMAL
          en:state_EngineSpeed = NORMAL;
        SENSOR.NORMAL.NORMAL.DEBOUNCE -> SENSOR.NORMAL.NORMAL.NORMAL : [(debounceCount >= CD_ENGINE_SPEED_DEBOUNCE_NORMAL)...
            | || (state_EngineSpeed == NORMAL)]
        (default) -> SENSOR.NORMAL.NORMAL.DEBOUNCE
      note: We check sensor supply 2 as EOP runs off that voltage, if it is in error
          | the EOP will not report back a valid reading.
      state NO_SIGNAL
        state DEBOUNCE
          en:debounceCount = 0;
          du:debounceCount++;
        state NO_SIGNAL
          en:state_EngineSpeed = NO_SIGNAL;
        SENSOR.NORMAL.NO_SIGNAL.DEBOUNCE -> SENSOR.NORMAL.NO_SIGNAL.NO_SIGNAL : [(debounceCount >= CD_ENGINE_SPEED_DEBOUNCE_NO_SIGNAL)...
            | || (state_EngineSpeed == NO_SIGNAL)]
        (default) -> SENSOR.NORMAL.NO_SIGNAL.DEBOUNCE
      SENSOR.NORMAL.SHUTDOWN -> SENSOR.NORMAL.EXTREMELY_HIGH : [(state_EngineSpeed != SHUTDOWN)...
          | && (flt_EngineSpeed_in < CD_ENGINE_SPEED_EXTREMELY_HIGH)]
      SENSOR.NORMAL.EXTREMELY_HIGH -> SENSOR.NORMAL.SHUTDOWN [order 2] : [(CD_SHUTDOWN_FUNCTION != NON_FUNCTIONAL)...
          | && (state_EngineSpeed == EXTREMELY_HIGH)]
      SENSOR.NORMAL.EXTREMELY_HIGH -> SENSOR.NORMAL.HIGH [order 1] : [(flt_EngineSpeed_in < CD_ENGINE_SPEED_EXTREMELY_HIGH)]
      SENSOR.NORMAL.HIGH -> SENSOR.NORMAL.EXTREMELY_HIGH [order 1] : [(flt_EngineSpeed_in >= CD_ENGINE_SPEED_EXTREMELY_HIGH)]
      SENSOR.NORMAL.HIGH -> SENSOR.NORMAL.NORMAL [order 2] : [(flt_EngineSpeed_in < CD_ENGINE_SPEED_HIGH)]
      SENSOR.NORMAL.NORMAL -> SENSOR.NORMAL.HIGH [order 2] : [(flt_EngineSpeed_in >= CD_ENGINE_SPEED_HIGH)]
      (default) -> SENSOR.NORMAL.NORMAL
      SENSOR.NORMAL.NO_SIGNAL -> SENSOR.NORMAL.NORMAL : [(flt_EngineSpeed_in > CD_ENGINE_SPEED_NO_SIGNAL)...
          | || (state_EOP != NORMAL)...
          | || (state_SensorSupply2 != NORMAL)...
          | || (((CD_EOP_FUNCTION != SWITCH_INPUT) && (flt_EOP < CD_EOP_NO_ENGINE_SPEED_SIGNAL_VALUE))...
          |     || ((CD_EOP_FUNCTION == SWITCH_INPUT) && (adin_EOP <= CD_EOP_SWITCH_LOW)))]
      SENSOR.NORMAL.NORMAL -> SENSOR.NORMAL.NO_SIGNAL [order 1] : [(flt_EngineSpeed_in <= CD_ENGINE_SPEED_NO_SIGNAL)...
          | && (state_EOP == NORMAL)...
          | && (state_SensorSupply2 == NORMAL)...
          | &&...
          | (((CD_EOP_FUNCTION != SWITCH_INPUT)  && (state_EOP == NORMAL) && (flt_EOP >= CD_EOP_NO_ENGINE_SPEED_SIGNAL_VALUE))...
          |  || ((CD_EOP_FUNCTION == SWITCH_INPUT) && (adin_EOP > CD_EOP_SWITCH_LOW)))]
    state NON_FUNCTIONAL
      en:state_EngineSpeed = NORMAL;
    SENSOR.OUT_OF_RANGE -> SENSOR.NORMAL : [(flt_EngineSpeed_in < CD_ENGINE_SPEED_OUT_OF_RANGE)]
    SENSOR.NORMAL -> SENSOR.OUT_OF_RANGE [order 1] : [(flt_EngineSpeed_in >= CD_ENGINE_SPEED_OUT_OF_RANGE)]
    NON_FUNCTIONAL -> SENSOR.NORMAL : [(CD_ENGINE_SPEED_FUNCTION != NON_FUNCTIONAL)...
        | && (state_System == SYS_NORMAL)...
        | && (CD_ECU_FUNCTION == NON_FUNCTIONAL)]
    SENSOR.NORMAL -> NON_FUNCTIONAL [order 2] : [(state_System != SYS_NORMAL)]
    (default) -> NON_FUNCTIONAL
  state ECU
    state NORMAL
      du:flt_EngineSpeed_out = flt_EngineSpeed_in;
      state NORMAL
        en:state_EngineSpeed = NORMAL;
      state INVALID_DATA
        du:flt_EngineSpeed_out = flt_EngineSpeed_in;
        state FAULT
          en:state_EngineSpeed = INVALID_DATA;
        state DEBOUNCE
          en:debounceCount = 0;
          du:debounceCount++;
        (default) -> ECU.NORMAL.INVALID_DATA.DEBOUNCE
        ECU.NORMAL.INVALID_DATA.DEBOUNCE -> FAULT : [(debounceCount >= CD_ENGINE_SPEED_DEBOUNCE_INVALID_DATA)...
            | || (state_EngineSpeed == INVALID_DATA)]
      (default) -> ECU.NORMAL.NORMAL
      ECU.NORMAL.NORMAL -> INVALID_DATA : [(CD_ECU_FUNCTION == ECU_KUBOTA)...
          | && (state_System == SYS_NORMAL)...
          | && (state_CommECU == NORMAL)...
          | && ((ecu_isocMaxRPM <= CD_ECU_MAX_ENGINE_SPEED_LOW)...
          |        || (ecu_isocMaxRPM >= CD_ECU_MAX_ENGINE_SPEED_HIGH)...
          |        || (ecu_isocMinRPM <= CD_ECU_MIN_ENGINE_SPEED_LOW)...
          |        || (ecu_isocMinRPM >= CD_ECU_MIN_ENGINE_SPEED_HIGH))]
    state NO_COMMUNICATION
      en: flt_EngineSpeed_out = 0;
    NO_COMMUNICATION -> ECU.NORMAL : [(state_CommECU != NO_COMMUNICATION)]
    (default) -> ECU.NORMAL
    ECU.NORMAL -> NO_COMMUNICATION : [(state_CommECU == NO_COMMUNICATION)]
  (default) -> SENSOR
  SENSOR -> ECU : [(CD_ECU_FUNCTION != NON_FUNCTIONAL)]
  data: debounceCount local uint16; flt_EngineSpeed_in input uint16; state_EOP input uint8; state_EngineSpeed output uint8; flt_EOP input uint16; CD_ENGINE_SPEED_FUNCTION parameter uint8; CD_ENGINE_SPEED_NO_SIGNAL parameter uint16; CD_ENGINE_SPEED_HIGH parameter uint16; CD_ENGINE_SPEED_EXTREMELY_HIGH parameter uint16; CD_ENGINE_SPEED_DEBOUNCE_NORMAL parameter uint16; CD_ENGINE_SPEED_DEBOUNCE_HIGH parameter uint16; CD_ENGINE_SPEED_DEBOUNCE_EXTREMELY_HIGH parameter uint16; CD_EOP_NO_ENGINE_SPEED_SIGNAL_VALUE parameter uint8; CD_ENGINE_SPEED_DEBOUNCE_NO_SIGNAL parameter uint16; CD_ENGINE_SPEED_DEBOUNCE_OUT_OF_RANGE parameter uint16; CD_ENGINE_SPEED_OUT_OF_RANGE parameter uint16; CD_ENGINE_SPEED_DEBOUNCE_SHUTDOWN parameter uint16; CD_SHUTDOWN_FUNCTION parameter uint8; HIGH parameter uint8 =10; EXTREMELY_HIGH parameter uint8 =11; NO_SIGNAL parameter uint8 =13; SHUTDOWN parameter uint8 =15; OUT_OF_RANGE parameter uint8 =18; NON_FUNCTIONAL parameter uint8 =255; NORMAL parameter uint8 =8; CD_EOP_FUNCTION parameter uint8; state_System input uint8; SYS_NORMAL parameter uint8; adin_EOP input uint16; CD_EOP_SWITCH_LOW parameter uint16; SWITCH_INPUT parameter uint8; CD_ECU_FUNCTION parameter uint8; state_CommECU input uint8; NO_COMMUNICATION parameter uint8; state_SensorSupply2 input uint8; flt_EngineSpeed_out output uint16; CD_ECU_MAX_ENGINE_SPEED_HIGH parameter uint16; CD_ECU_MAX_ENGINE_SPEED_LOW parameter uint16; CD_ECU_MIN_ENGINE_SPEED_HIGH parameter uint16; CD_ECU_MIN_ENGINE_SPEED_LOW parameter uint16; CD_ENGINE_SPEED_DEBOUNCE_INVALID_DATA parameter uint16; ecu_isocMaxRPM input uint16; ecu_isocMinRPM input uint16; ECU_KUBOTA parameter uint8; INVALID_DATA parameter uint8
